simulink model "ExRobotAndEnvironmentController"  (Simulink 8.3)
settings: Solver=ode45  StartTime=0.0  StopTime=1000  FixedStep=.01  RelTol=1e-3
undefined symbols (not defined in the file or in its folder): Env, INITIAL_ROBOT_POS_THETA, INITIAL_ROBOT_POS_X, INITIAL_ROBOT_POS_Y, INTER_WHEEL_DISTANCE, ki_teta, kp_teta, MAX_SPEED, Robot, RobotInit, ts, ts_anim
libraries: simulink x1
settings Model: Creator=alex  LastModifiedBy=elkhadiy
settings OptimizationCC: ExpressionDepthLimit=2147483647
settings DebuggingCC: SolverPrmCheckMsg=none  FcnCallInpInsideContextMsg=UseLocalSettings
settings SFSimCC: SimParseCustomCode=off

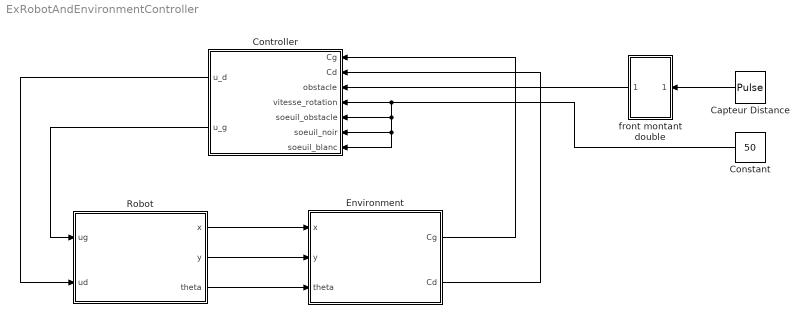
== system ExRobotAndEnvironmentController ==
  Capteur Distance : DiscretePulseGenerator  PulseType=Time based  Amplitude=100  Period=5  PulseWidth=5  PhaseDelay=3
  Constant : Constant  Value=50
  Controller : Subsystem
  Environment : Subsystem
  Robot : Subsystem
  front montant double : Subsystem
  wires:
  Robot/1(x) -> Environment/1(x)
  Robot/2(y) -> Environment/2(y)
  Robot/3(theta) -> Environment/3(theta)
  Environment/1(Cg) -> Controller/1(Cg)
  Environment/2(Cd) -> Controller/2(Cd)
  Controller/1(u_d) -> Robot/2(ud)
  Controller/2(u_g) -> Robot/1(ug)
  front montant double/1(Out1) -> Controller/3(obstacle)
  Capteur Distance/1 -> front montant double/1(In1)
  Constant/1 -> Controller/7(soeuil_blanc), Controller/6(soeuil_noir), Controller/5(soeuil_obstacle), Controller/4(vitesse_rotation)

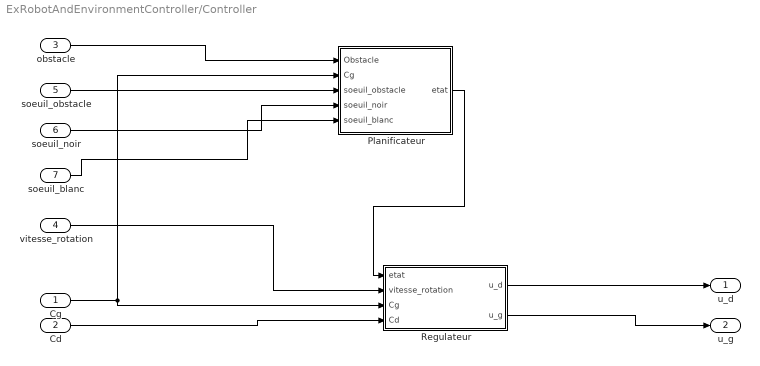
== system ExRobotAndEnvironmentController/Controller ==
  Cg : Inport  OutDataTypeStr=double
  Cd : Inport  Port=2  OutDataTypeStr=double
  obstacle : Inport  Port=3  OutDataTypeStr=double
  vitesse_rotation : Inport  Port=4  OutDataTypeStr=double
  soeuil_obstacle : Inport  Port=5  OutDataTypeStr=double
  soeuil_noir : Inport  Port=6  OutDataTypeStr=double
  soeuil_blanc : Inport  Port=7  OutDataTypeStr=double
  Planificateur : Subsystem
  Regulateur : Subsystem
  u_d : Outport
  u_g : Outport  Port=2
  wires:
  Cg/1 -> Regulateur/3(Cg), Planificateur/2(Cg)
  obstacle/1 -> Planificateur/1(Obstacle)
  soeuil_obstacle/1 -> Planificateur/3(soeuil_obstacle)
  soeuil_noir/1 -> Planificateur/4(soeuil_noir)
  soeuil_blanc/1 -> Planificateur/5(soeuil_blanc)
  Planificateur/1(etat) -> Regulateur/1(etat)
  vitesse_rotation/1 -> Regulateur/2(vitesse_rotation)
  Cd/1 -> Regulateur/4(Cd)
  Regulateur/1(u_d) -> u_d/1
  Regulateur/2(u_g) -> u_g/1

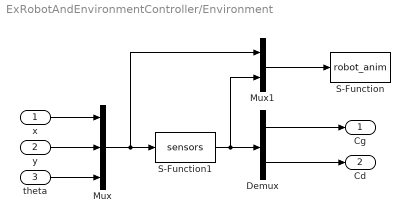
== system ExRobotAndEnvironmentController/Environment ==
  x : Inport
  y : Inport  Port=2
  theta : Inport  Port=3
  Demux : Demux  Outputs=2
  Mux : Mux  Inputs=3
  Mux1 : Mux  Inputs=2
  S-Function : S-Function  FunctionName=robot_anim  Parameters=ts_anim,Env,Robot,RobotInit  EnableBusSupport=off
  S-Function1 : S-Function  FunctionName=sensors  Parameters=ts,Env,Robot  EnableBusSupport=off
  Cg : Outport
  Cd : Outport  Port=2
  wires:
  x/1 -> Mux/1
  y/1 -> Mux/2
  theta/1 -> Mux/3
  Mux/1 -> S-Function1/1, Mux1/1
  S-Function1/1 -> Mux1/2, Demux/1
  Mux1/1 -> S-Function/1
  Demux/1 -> Cg/1
  Demux/2 -> Cd/1

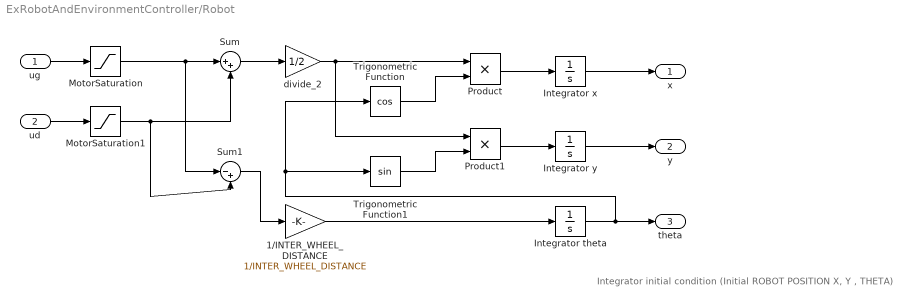
== system ExRobotAndEnvironmentController/Robot ==
  note: Integrator initial condition (Initial ROBOT POSITION X, Y , THETA)
  ug : Inport
  ud : Inport  Port=2
  1/INTER_WHEEL_DISTANCE : Gain  Gain=1/INTER_WHEEL_DISTANCE
  Integrator theta : Integrator  InitialCondition=INITIAL_ROBOT_POS_THETA
  Integrator x : Integrator  InitialCondition=INITIAL_ROBOT_POS_X
  Integrator y : Integrator  InitialCondition=INITIAL_ROBOT_POS_Y
  MotorSaturation : Saturate  UpperLimit=MAX_SPEED  LowerLimit=-MAX_SPEED
  MotorSaturation1 : Saturate  UpperLimit=MAX_SPEED  LowerLimit=-MAX_SPEED
  Product : Product  RndMeth=Zero
  Product1 : Product  RndMeth=Zero
  Sum : Sum  Inputs=|++
  Sum1 : Sum  Inputs=|-+
  Trigonometric Function : Trigonometry  Operator=cos
  Trigonometric Function1 : Trigonometry
  divide_2 : Gain  Gain=1/2
  x : Outport
  y : Outport  Port=2
  theta : Outport  Port=3
  wires:
  ug/1 -> MotorSaturation/1
  Integrator x/1 -> x/1
  Integrator y/1 -> y/1
  Integrator theta/1 -> Trigonometric Function/1, Trigonometric Function1/1, theta/1
  Sum/1 -> divide_2/1
  divide_2/1 -> Product1/1, Product/1
  Trigonometric Function/1 -> Product/2
  Trigonometric Function1/1 -> Product1/2
  Product/1 -> Integrator x/1
  Product1/1 -> Integrator y/1
  Sum1/1 -> 1/INTER_WHEEL_DISTANCE/1
  1/INTER_WHEEL_DISTANCE/1 -> Integrator theta/1
  ud/1 -> MotorSaturation1/1
  MotorSaturation1/1 -> Sum/2, Sum1/2
  MotorSaturation/1 -> Sum/1, Sum1/1

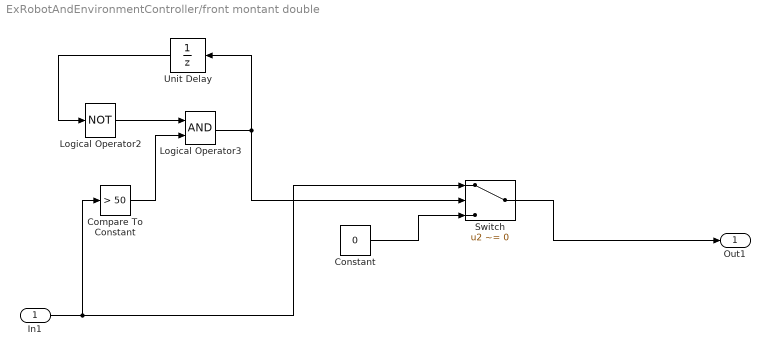
== system ExRobotAndEnvironmentController/front montant double ==
  In1 : Inport
  Compare To Constant : simulink/Logic and Bit Operations/Compare To Constant  relop=>  const=50  OutDataTypeStr=boolean
  Constant : Constant  Value=0
  Logical Operator2 : Logic  Operator=NOT  AllPortsSameDT=off  OutDataTypeStr=boolean
  Logical Operator3 : Logic  AllPortsSameDT=off  OutDataTypeStr=boolean
  Switch : Switch  Criteria=u2 ~= 0
  Unit Delay : UnitDelay  SampleTime=-1
  Out1 : Outport  OutDataTypeStr=double
  wires:
  Logical Operator2/1 -> Logical Operator3/1
  Unit Delay/1 -> Logical Operator2/1
  Compare To Constant/1 -> Logical Operator3/2
  Logical Operator3/1 -> Unit Delay/1, Switch/2
  In1/1 -> Switch/1, Compare To Constant/1
  Switch/1 -> Out1/1
  Constant/1 -> Switch/3

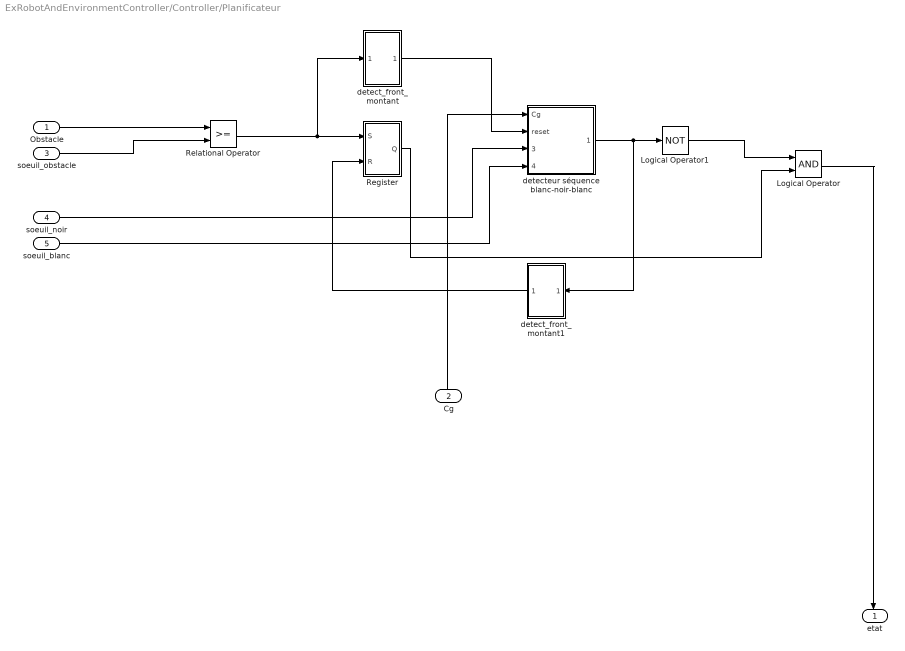
== system ExRobotAndEnvironmentController/Controller/Planificateur ==
  Obstacle : Inport  OutDataTypeStr=double
  Cg : Inport  Port=2  OutDataTypeStr=double
  soeuil_obstacle : Inport  Port=3  OutDataTypeStr=double
  soeuil_noir : Inport  Port=4  OutDataTypeStr=double
  soeuil_blanc : Inport  Port=5  OutDataTypeStr=double
  Logical Operator : Logic  AllPortsSameDT=off  OutDataTypeStr=boolean
  Logical Operator1 : Logic  Operator=NOT  AllPortsSameDT=off  OutDataTypeStr=boolean
  Register : Subsystem
  Relational Operator : RelationalOperator  OutDataTypeStr=boolean
  detect_front_montant : Subsystem
  detect_front_montant1 : Subsystem
  detecteur séquence blanc-noir-blanc : Subsystem
  etat : Outport
  wires:
  detect_front_montant/1(Out1) -> detecteur séquence blanc-noir-blanc/2(reset)
  Cg/1 -> detecteur séquence blanc-noir-blanc/1(Cg)
  Logical Operator1/1 -> Logical Operator/1
  Relational Operator/1 -> detect_front_montant/1(In1), Register/1(S)
  detect_front_montant1/1(Out1) -> Register/2(R)
  Register/1(Q) -> Logical Operator/2
  detecteur séquence blanc-noir-blanc/1(séquence repérée) -> detect_front_montant1/1(In1), Logical Operator1/1
  Logical Operator/1 -> etat/1
  soeuil_obstacle/1 -> Relational Operator/2
  Obstacle/1 -> Relational Operator/1
  soeuil_noir/1 -> detecteur séquence blanc-noir-blanc/3(soeuil_noir)
  soeuil_blanc/1 -> detecteur séquence blanc-noir-blanc/4(soeuil_blanc)

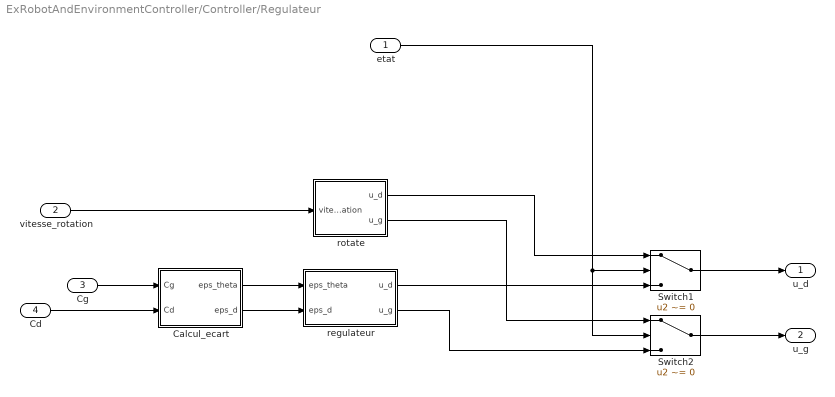
== system ExRobotAndEnvironmentController/Controller/Regulateur ==
  etat : Inport  OutDataTypeStr=boolean
  vitesse_rotation : Inport  Port=2  OutDataTypeStr=double
  Cg : Inport  Port=3  OutDataTypeStr=double
  Cd : Inport  Port=4  OutDataTypeStr=double
  Calcul_ecart : Subsystem
  Switch1 : Switch  Criteria=u2 ~= 0
  Switch2 : Switch  Criteria=u2 ~= 0
  regulateur : Subsystem
  rotate : Subsystem
  u_d : Outport
  u_g : Outport  Port=2
  wires:
  etat/1 -> Switch2/2, Switch1/2
  Cg/1 -> Calcul_ecart/1(Cg)
  vitesse_rotation/1 -> rotate/1(vitesse_rotation)
  Calcul_ecart/2(eps_d) -> regulateur/2(eps_d)
  Cd/1 -> Calcul_ecart/2(Cd)
  Calcul_ecart/1(eps_theta) -> regulateur/1(eps_theta)
  Switch1/1 -> u_d/1
  Switch2/1 -> u_g/1
  regulateur/1(u_d) -> Switch1/3
  regulateur/2(u_g) -> Switch2/3
  rotate/2(u_g) -> Switch2/1
  rotate/1(u_d) -> Switch1/1

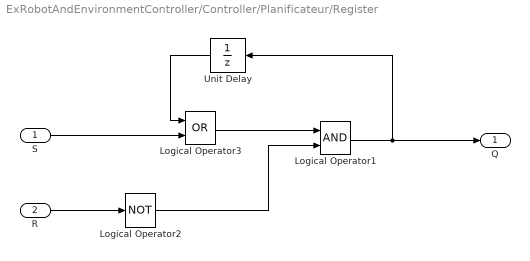
== system ExRobotAndEnvironmentController/Controller/Planificateur/Register ==
  S : Inport
  R : Inport  Port=2
  Logical Operator1 : Logic  AllPortsSameDT=off  OutDataTypeStr=boolean
  Logical Operator2 : Logic  Operator=NOT  AllPortsSameDT=off  OutDataTypeStr=boolean
  Logical Operator3 : Logic  Operator=OR  AllPortsSameDT=off  OutDataTypeStr=boolean
  Unit Delay : UnitDelay  SampleTime=-1
  Q : Outport
  wires:
  Logical Operator1/1 -> Unit Delay/1, Q/1
  Unit Delay/1 -> Logical Operator3/1
  Logical Operator2/1 -> Logical Operator1/2
  Logical Operator3/1 -> Logical Operator1/1
  S/1 -> Logical Operator3/2
  R/1 -> Logical Operator2/1

== system ExRobotAndEnvironmentController/Controller/Planificateur/detect_front_montant ==
  In1 : Inport
  Logical Operator2 : Logic  Operator=NOT  AllPortsSameDT=off  OutDataTypeStr=boolean
  Logical Operator3 : Logic  AllPortsSameDT=off  OutDataTypeStr=boolean
  Unit Delay : UnitDelay  SampleTime=-1
  Out1 : Outport
  wires:
  In1/1 -> Unit Delay/1, Logical Operator3/2
  Logical Operator2/1 -> Logical Operator3/1
  Unit Delay/1 -> Logical Operator2/1
  Logical Operator3/1 -> Out1/1

== system ExRobotAndEnvironmentController/Controller/Planificateur/detect_front_montant1 ==
  In1 : Inport
  Logical Operator2 : Logic  Operator=NOT  AllPortsSameDT=off  OutDataTypeStr=boolean
  Logical Operator3 : Logic  AllPortsSameDT=off  OutDataTypeStr=boolean
  Unit Delay : UnitDelay  SampleTime=-1
  Out1 : Outport
  wires:
  In1/1 -> Unit Delay/1, Logical Operator3/2
  Logical Operator2/1 -> Logical Operator3/1
  Unit Delay/1 -> Logical Operator2/1
  Logical Operator3/1 -> Out1/1

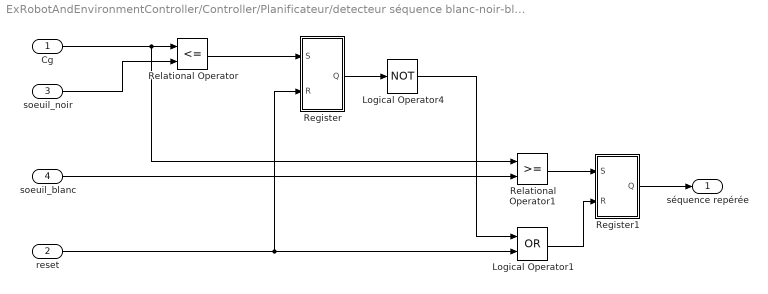
== system ExRobotAndEnvironmentController/Controller/Planificateur/detecteur séquence blanc-noir-blanc ==
  Cg : Inport
  reset : Inport  Port=2  OutDataTypeStr=boolean
  soeuil_noir : Inport  Port=3
  soeuil_blanc : Inport  Port=4
  Logical Operator1 : Logic  Operator=OR  AllPortsSameDT=off  OutDataTypeStr=boolean
  Logical Operator4 : Logic  Operator=NOT  AllPortsSameDT=off  OutDataTypeStr=boolean
  Register : Subsystem
  Register1 : Subsystem
  Relational Operator : RelationalOperator  Operator=<=  OutDataTypeStr=boolean
  Relational Operator1 : RelationalOperator  OutDataTypeStr=boolean
  séquence repérée : Outport  OutDataTypeStr=boolean
  wires:
  Logical Operator4/1 -> Logical Operator1/1
  reset/1 -> Register/2(R), Logical Operator1/2
  Register/1(Q) -> Logical Operator4/1
  Relational Operator/1 -> Register/1(S)
  Relational Operator1/1 -> Register1/1(S)
  Logical Operator1/1 -> Register1/2(R)
  Cg/1 -> Relational Operator1/1, Relational Operator/1
  Register1/1(Q) -> séquence repérée/1
  soeuil_noir/1 -> Relational Operator/2
  soeuil_blanc/1 -> Relational Operator1/2

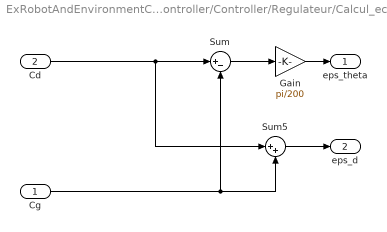
== system ExRobotAndEnvironmentController/Controller/Regulateur/Calcul_ecart ==
  Cg : Inport
  Cd : Inport  Port=2
  Gain : Gain  Gain=pi/200
  Sum : Sum  Inputs=|+-
  Sum5 : Sum  Inputs=|++
  eps_theta : Outport
  eps_d : Outport  Port=2
  wires:
  Sum/1 -> Gain/1
  Cd/1 -> Sum/1, Sum5/1
  Cg/1 -> Sum/2, Sum5/2
  Gain/1 -> eps_theta/1
  Sum5/1 -> eps_d/1

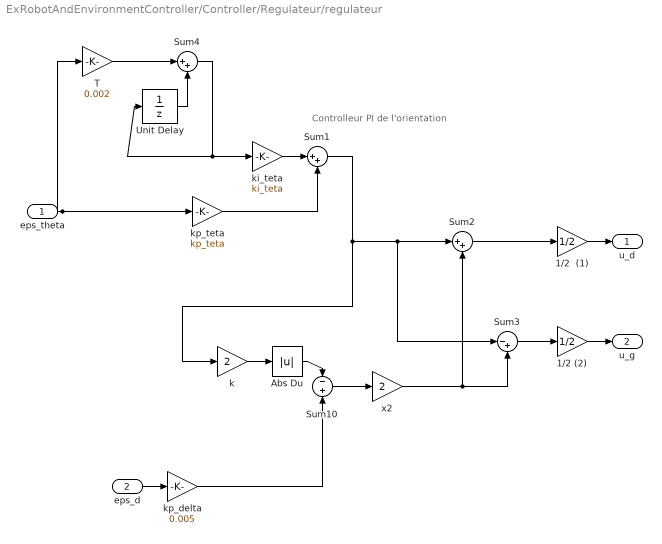
== system ExRobotAndEnvironmentController/Controller/Regulateur/regulateur ==
  note: Controlleur PI de l'orientation
  eps_theta : Inport
  eps_d : Inport  Port=2
  1/2  (1) : Gain  Gain=1/2  SaturateOnIntegerOverflow=on  OutDataTypeStr=Inherit: Same as input  ParamDataTypeStr=Inherit: Same as input
  1/2 (2) : Gain  Gain=1/2  SaturateOnIntegerOverflow=on  OutDataTypeStr=Inherit: Same as input  ParamDataTypeStr=Inherit: Same as input
  Abs Du : Abs  SaturateOnIntegerOverflow=on
  Sum1 : Sum  Inputs=|++  SaturateOnIntegerOverflow=on
  Sum10 : Sum  Inputs=-+  SaturateOnIntegerOverflow=on
  Sum2 : Sum  Inputs=|++  SaturateOnIntegerOverflow=on
  Sum3 : Sum  Inputs=|-+  SaturateOnIntegerOverflow=on
  Sum4 : Sum  Inputs=|++
  T : Gain  Gain=0.002
  Unit Delay : UnitDelay  SampleTime=-1
  k : Gain  Gain=2  SaturateOnIntegerOverflow=on  OutDataTypeStr=Inherit: Same as input  ParamDataTypeStr=Inherit: Same as input
  ki_teta : Gain  Gain=ki_teta  SaturateOnIntegerOverflow=on  OutDataTypeStr=Inherit: Same as input  ParamDataTypeStr=Inherit: Same as input
  kp_delta : Gain  Gain=0.005
  kp_teta : Gain  Gain=kp_teta  SaturateOnIntegerOverflow=on  OutDataTypeStr=Inherit: Same as input  ParamDataTypeStr=Inherit: Same as input
  x2 : Gain  Gain=2  SaturateOnIntegerOverflow=on  OutDataTypeStr=Inherit: Same as input  ParamDataTypeStr=Inherit: Same as input
  u_d : Outport
  u_g : Outport  Port=2
  wires:
  ki_teta/1 -> Sum1/1
  kp_teta/1 -> Sum1/2
  Sum2/1 -> 1/2  (1)/1
  Sum3/1 -> 1/2 (2)/1
  k/1 -> Abs Du/1
  kp_delta/1 -> Sum10/2
  eps_theta/1 -> kp_teta/1, T/1
  Abs Du/1 -> Sum10/1
  x2/1 -> Sum2/2, Sum3/2
  Sum10/1 -> x2/1
  Sum1/1 -> k/1, Sum2/1, Sum3/1
  T/1 -> Sum4/1
  Sum4/1 -> ki_teta/1, Unit Delay/1
  Unit Delay/1 -> Sum4/2
  1/2  (1)/1 -> u_d/1
  1/2 (2)/1 -> u_g/1
  eps_d/1 -> kp_delta/1

== system ExRobotAndEnvironmentController/Controller/Regulateur/rotate ==
  vitesse_rotation : Inport
  Gain : Gain  Gain=-1
  u_d : Outport
  u_g : Outport  Port=2
  wires:
  Gain/1 -> u_g/1
  vitesse_rotation/1 -> Gain/1, u_d/1

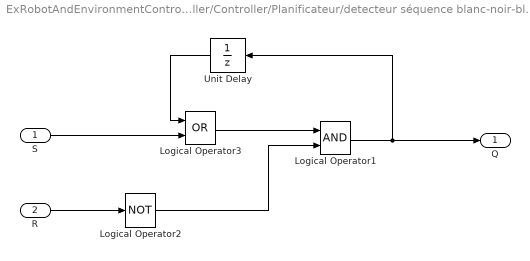
== system ExRobotAndEnvironmentController/Controller/Planificateur/detecteur séquence blanc-noir-blanc/Register ==
  S : Inport  OutDataTypeStr=boolean
  R : Inport  Port=2  OutDataTypeStr=boolean
  Logical Operator1 : Logic  AllPortsSameDT=off  OutDataTypeStr=boolean
  Logical Operator2 : Logic  Operator=NOT  AllPortsSameDT=off  OutDataTypeStr=boolean
  Logical Operator3 : Logic  Operator=OR  AllPortsSameDT=off  OutDataTypeStr=boolean
  Unit Delay : UnitDelay  SampleTime=-1
  Q : Outport
  wires:
  Logical Operator1/1 -> Unit Delay/1, Q/1
  Unit Delay/1 -> Logical Operator3/1
  Logical Operator2/1 -> Logical Operator1/2
  Logical Operator3/1 -> Logical Operator1/1
  S/1 -> Logical Operator3/2
  R/1 -> Logical Operator2/1

== system ExRobotAndEnvironmentController/Controller/Planificateur/detecteur séquence blanc-noir-blanc/Register1 ==
  S : Inport  OutDataTypeStr=boolean
  R : Inport  Port=2  OutDataTypeStr=boolean
  Logical Operator1 : Logic  AllPortsSameDT=off  OutDataTypeStr=boolean
  Logical Operator2 : Logic  Operator=NOT  AllPortsSameDT=off  OutDataTypeStr=boolean
  Logical Operator3 : Logic  Operator=OR  AllPortsSameDT=off  OutDataTypeStr=boolean
  Unit Delay : UnitDelay  SampleTime=-1
  Q : Outport
  wires:
  Logical Operator1/1 -> Unit Delay/1, Q/1
  Unit Delay/1 -> Logical Operator3/1
  Logical Operator2/1 -> Logical Operator1/2
  Logical Operator3/1 -> Logical Operator1/1
  S/1 -> Logical Operator3/2
  R/1 -> Logical Operator2/1
